simulink model "hw2"  (R2025b)
settings: Solver=VariableStepAuto  StartTime=0.0  StopTime=10.0  RelTol=1e-3
settings Model: Creator=elija  LastModifiedBy=elija

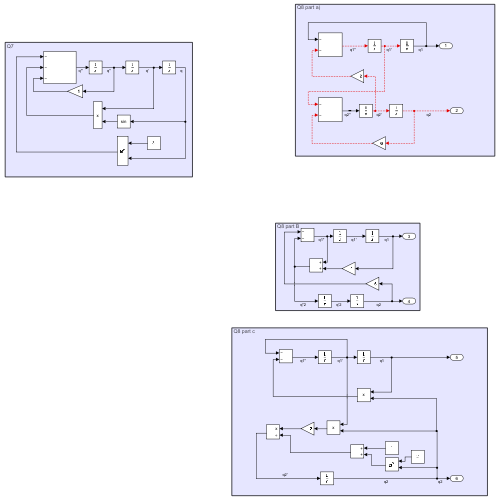
[thumbnail: Simulink's stored preview of the top-level diagram]
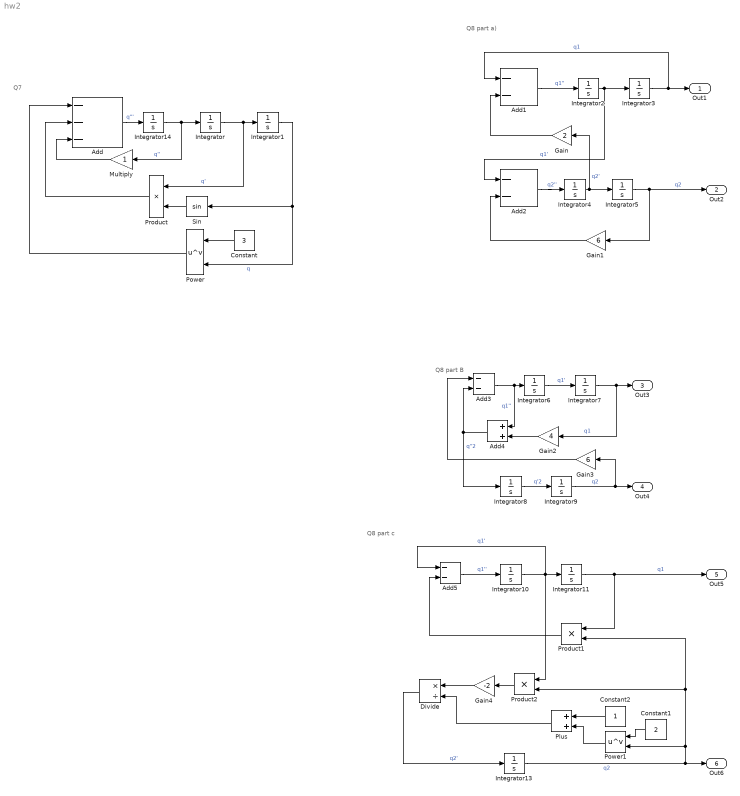
== system hw2 ==
  note: Q8 part c
  note: Q8 part B
  note: Q8 part a)
  note: Q7
  Add : Sum  Inputs=---
  Add{1..3,5} (4 alike) : Sum  Inputs=--
  Add4 : Sum
  Constant : Constant  Value=3
  Constant1 : Constant  Value=2
  Constant2 : Constant
  Divide : Product  Inputs=*/
  Gain : Gain  Gain=2
  Gain1 : Gain  Gain=6
  Gain2 : Gain  Gain=4
  Gain3 : Gain  Gain=6
  Gain4 : Gain  Gain=-2
  Integrator{,1..11,13..14} (14 alike) : Integrator
  Multiply : Gain
  Plus : Sum
  Power : Math  Operator=pow
  Power1 : Math  Operator=pow
  Product : Product
  Product1 : Product
  Product2 : Product
  Sin : Trigonometry
  Out1 : Outport
  Out2 : Outport  Port=2  VectorParamsAs1DForOutWhenUnconnected=off
  Out3 : Outport  Port=3
  Out4 : Outport  Port=4
  Out5 : Outport  Port=5
  Out6 : Outport  Port=6
  wires:
  Integrator/1 -> Product/1, Integrator1/1  "q'"
  Integrator1/1 -> Sin/1, Power/2  "q"
  Constant/1 -> Power/1
  Power/1 -> Add/1
  Sin/1 -> Product/2
  Product/1 -> Add/2
  Multiply/1 -> Add/3
  Add1/1 -> Integrator2/1  "q1''"
  Integrator2/1 -> Integrator3/1, Add2/1  "q1'"
  Integrator3/1 -> Out1/1, Add1/1  "q1"
  Add2/1 -> Integrator4/1  "q2''"
  Integrator4/1 -> Gain/1, Integrator5/1  "q2'"
  Integrator5/1 -> Gain1/1, Out2/1  "q2"
  Gain/1 -> Add1/2
  Gain1/1 -> Add2/2
  Integrator6/1 -> Integrator7/1  "q1'"
  Add3/1 -> Add4/1, Integrator6/1  "q1''"
  Integrator7/1 -> Gain2/1, Out3/1  "q1"
  Gain2/1 -> Add4/2
  Add4/1 -> Integrator8/1, Add3/2  "q''2"
  Integrator8/1 -> Integrator9/1  "q'2"
  Integrator9/1 -> Out4/1, Gain3/1  "q2"
  Gain3/1 -> Add3/1
  Add5/1 -> Integrator10/1  "q1''"
  Integrator10/1 -> Integrator11/1, Product2/1, Add5/1  "q1'"
  Integrator11/1 -> Product1/1, Out5/1  "q1"
  Product2/1 -> Gain4/1
  Gain4/1 -> Divide/1
  Product1/1 -> Add5/2
  Divide/1 -> Integrator13/1  "q2'"
  Integrator13/1 -> Out6/1, Product1/2, Product2/2, Power1/2  "q2"
  Power1/1 -> Plus/2
  Constant1/1 -> Power1/1
  Plus/1 -> Divide/2
  Constant2/1 -> Plus/1
  Add/1 -> Integrator14/1  "q'''"
  Integrator14/1 -> Multiply/1, Integrator/1  "q''"
